simulink model "ThrustVectorControlModelRocket"  (R2018a)
settings: Solver=FixedStepAuto  StartTime=0.0  StopTime=3.5  FixedStep=0.02  RelTol=1e-3
libraries: simulink_extras x7, simulink x5, sharedtransform x1, aerolibutil x1
settings Model: Creator=Doe  LastModifiedBy=rahul
settings OptimizationCC: DefaultParameterBehavior=Inlined  UseDivisionForNetSlopeComputation=on  UseFloatMulNetSlope=on  InlineInvariantSignals=on  PassReuseOutputArgsAs=Individual arguments  ZeroExternalMemoryAtStartup=off  ZeroInternalMemoryAtStartup=off  NoFixptDivByZeroProtection=on  EfficientFloat2IntCast=on  LifeSpan=1  OptimizeBlockOrder=speed  DifferentSizesBufferReuse=on
settings DebuggingCC: ParameterTunabilityLossMsg=error
settings HardwareCC: ProdBitPerInt=16  ProdBitPerPointer=16  ProdBitPerSizeT=16  ProdBitPerPtrDiffT=16  ProdLargestAtomicFloat=None  ProdWordSize=16  ProdLongLongMode=on  ProdHWDeviceType=Atmel->AVR (8-bit)
settings SFSimCC: MATLABDynamicMemAlloc=off
settings RTWCC: SystemTargetFile=ert.tlc  TemplateMakefile=ert_default_tmf  GenerateReport=on  IncludeHyperlinkInReport=on  LaunchReport=on  TargetLang=C++  GenerateTraceInfo=on  GenerateTraceReport=on  GenerateTraceReportSl=on  GenerateTraceReportSf=on  GenerateTraceReportEml=on
settings CodeAppCC: ForceParamTrailComments=on  IgnoreCustomStorageClasses=off  OperatorAnnotations=on  SimulinkDataObjDesc=on  SFDataObjDesc=on  CustomSymbolStrGlobalVar=rt$N$M  CustomSymbolStrType=$N$M  CustomSymbolStrFcn=$N$M$F  CustomSymbolStrMacro=$N$M  InsertBlockDesc=on
settings ERTTargetCC: TargetLangStandard=C++03 (ISO)  GenerateSampleERTMain=on  IncludeMdlTerminateFcn=off  CombineSignalStateStructs=on  MultiInstanceERTCode=on  CodeInterfacePackaging=C++ class  SupportComplex=off  SupportContinuousTime=on  InlinedParameterPlacement=NonHierarchical  RootIOFormat=Structure reference  ERTCustomFileTemplate=example_file_process.tlc  ERTFilePackagingFormat=CompactWithDataFile

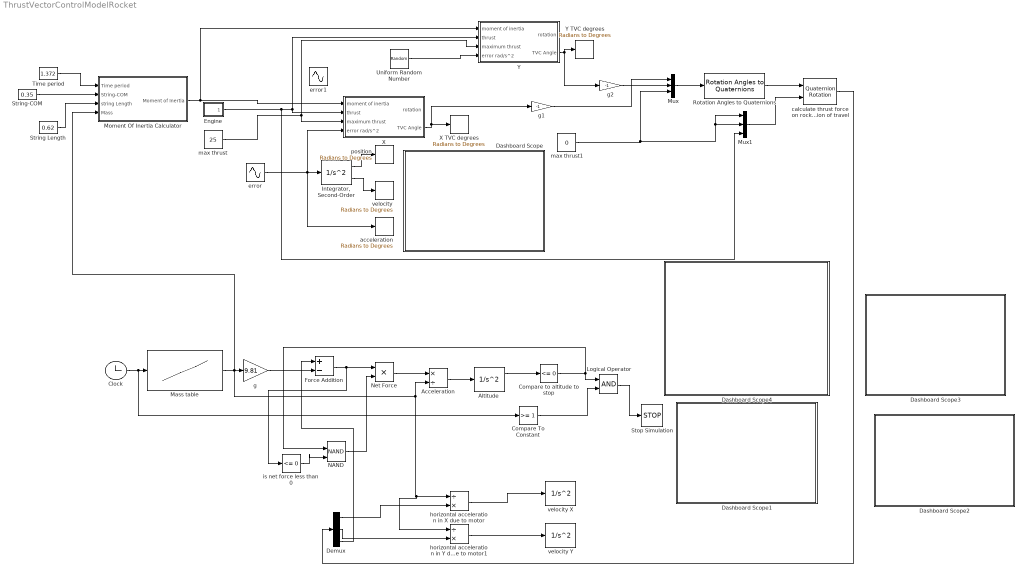
== system ThrustVectorControlModelRocket ==
  Acceleration : Product  Inputs=*/
  Altitude : SecondOrderIntegrator
  Clock : Clock
  Compare To Constant : simulink/Logic and Bit Operations/Compare To Constant  relop=>=  const=1  OutDataTypeStr=boolean
  Compare to altitude to stop : simulink/Logic and Bit Operations/Compare To Constant  relop=<=  const=0  OutDataTypeStr=boolean
  Dashboard Scope : Subsystem  DialogController=hmiCreateDDGDialog  IsWebBlock=on  mask(MWDashboardBlock){webBlockId=e89a2d5a-8c4b-4126-bd68-68e024a85c17, webBlockType=sdiscope, ShowInitialText=on, HMISrcModelName=ThrustVectorControlModelRocket}
      mask prompts: webBlockId "WebBlock Id"; webBlockType "WebBlock Type"; HMISrcModelName "Source Model"
      mask help: SimulinkHMI:dialogs:HMIScopeDialogDesc
      mask Help: helpview([docroot '/mapfiles/simulink.map'], 'hmi_scope')
      mask Display:
      | if strcmp(get_param(bdroot(gcb),'BlockDiagramType'), 'library')
      |     image([(matlabroot) '/toolbox/simulink/hmi/icons/DashboardScope.png']);
      | end
  Dashboard Scope1 : Subsystem  DialogController=hmiCreateDDGDialog  IsWebBlock=on  mask(MWDashboardBlock){webBlockId=79388a0e-acf4-4a0f-9f6d-7a65b6fe74ae, webBlockType=sdiscope, ShowInitialText=on, HMISrcModelName=ThrustVectorControlModelRocket}
      mask prompts: webBlockId "WebBlock Id"; webBlockType "WebBlock Type"; HMISrcModelName "Source Model"
      mask help: SimulinkHMI:dialogs:HMIScopeDialogDesc
      mask Help: helpview([docroot '/mapfiles/simulink.map'], 'hmi_scope')
      mask Display:
      | if strcmp(get_param(bdroot(gcb),'BlockDiagramType'), 'library')
      |     image([(matlabroot) '/toolbox/simulink/hmi/icons/DashboardScope.png']);
      | end
  Dashboard Scope2 : Subsystem  DialogController=hmiCreateDDGDialog  IsWebBlock=on  mask(MWDashboardBlock){webBlockId=9be5d186-43fb-46f6-9404-6296feed70e7, webBlockType=sdiscope, ShowInitialText=on, HMISrcModelName=ThrustVectorControlModelRocket}
      mask prompts: webBlockId "WebBlock Id"; webBlockType "WebBlock Type"; HMISrcModelName "Source Model"
      mask help: SimulinkHMI:dialogs:HMIScopeDialogDesc
      mask Help: helpview([docroot '/mapfiles/simulink.map'], 'hmi_scope')
      mask Display:
      | if strcmp(get_param(bdroot(gcb),'BlockDiagramType'), 'library')
      |     image([(matlabroot) '/toolbox/simulink/hmi/icons/DashboardScope.png']);
      | end
  Dashboard Scope3 : Subsystem  DialogController=hmiCreateDDGDialog  IsWebBlock=on  mask(MWDashboardBlock){webBlockId=200297c4-bc4f-4d0c-b2fb-30ef607173bc, webBlockType=sdiscope, ShowInitialText=on, HMISrcModelName=ThrustVectorControlModelRocket}
      mask prompts: webBlockId "WebBlock Id"; webBlockType "WebBlock Type"; HMISrcModelName "Source Model"
      mask help: SimulinkHMI:dialogs:HMIScopeDialogDesc
      mask Help: helpview([docroot '/mapfiles/simulink.map'], 'hmi_scope')
      mask Display:
      | if strcmp(get_param(bdroot(gcb),'BlockDiagramType'), 'library')
      |     image([(matlabroot) '/toolbox/simulink/hmi/icons/DashboardScope.png']);
      | end
  Dashboard Scope4 : Subsystem  DialogController=hmiCreateDDGDialog  IsWebBlock=on  mask(MWDashboardBlock){webBlockId=5d101f40-2dd7-4f18-8b35-aff23edb331a, webBlockType=sdiscope, ShowInitialText=on, HMISrcModelName=ThrustVectorControlModelRocket}
      mask prompts: webBlockId "WebBlock Id"; webBlockType "WebBlock Type"; HMISrcModelName "Source Model"
      mask help: SimulinkHMI:dialogs:HMIScopeDialogDesc
      mask Help: helpview([docroot '/mapfiles/simulink.map'], 'hmi_scope')
      mask Display:
      | if strcmp(get_param(bdroot(gcb),'BlockDiagramType'), 'library')
      |     image([(matlabroot) '/toolbox/simulink/hmi/icons/DashboardScope.png']);
      | end
  Demux : Demux  Outputs=3
  Engine : Subsystem
  Force Addition : Sum  Inputs=+-
  "Integrator, Second-Order" : SecondOrderIntegrator
  Logical Operator : Logic  AllPortsSameDT=off  OutDataTypeStr=boolean
  Mass table : Lookup  InputValues=[0,1]  Table=[0.975,.8]  LookUpMeth=Use Input Nearest  SaturateOnIntegerOverflow=on
  Moment Of Inertia Calculator : Subsystem
  Mux : Mux  Inputs=3
  Mux1 : Mux  Inputs=3
  NAND : Logic  Operator=NAND  IconShape=distinctive  AllPortsSameDT=off  OutDataTypeStr=boolean
  Net Force : Product  Inputs=**
  Rotation Angles to Quaternions : sharedtransform/Rotation Angles to Quaternions  rotationOrder=XYZ  aMode=aMode
      settings: SourceProductName=Aerospace Blockset  SourceProductBaseCode=AE
  Stop Simulation : Stop
  String Length : Constant  Value=0.62
  String-COM : Constant  Value=0.35
  Time period : Constant  Value=1.372
  Uniform Random Number : UniformRandomNumber  Minimum=-3  Maximum=3  SampleTime=.4
  X : Subsystem
  X TVC degrees : simulink_extras/Transformations/Radians to Degrees
  Y : Subsystem
  Y TVC degrees : simulink_extras/Transformations/Radians to Degrees
  acceleration : simulink_extras/Transformations/Radians to Degrees
  calculate thrust force on rocket in direction of travel : aerolibutil/Quaternion Rotation
  error : Sin  Amplitude=2  Frequency=2  SampleTime=0
  error1 : Sin  Frequency=4  SampleTime=0
  g : Gain  Gain=9.81
  g1 : Gain  Gain=-1
  g2 : Gain  Gain=-1
  horizontal acceleration in X due to motor : Product  Inputs=/*
  horizontal acceleration in Y due to motor1 : Product  Inputs=/*
  is net force less than 0 : simulink/Logic and Bit Operations/Compare To Constant  relop=<=  const=0  OutDataTypeStr=boolean
  max thrust : Constant  Value=25
  max thrust1 : Constant  Value=0
  position : simulink_extras/Transformations/Radians to Degrees
  velocity : simulink_extras/Transformations/Radians to Degrees
  velocity X : SecondOrderIntegrator
  velocity Y : SecondOrderIntegrator
  wires:
  String-COM/1 -> Moment Of Inertia Calculator/2(String-COM)
  Time period/1 -> Moment Of Inertia Calculator/1(Time period)
  String Length/1 -> Moment Of Inertia Calculator/3(string Length)
  NAND/1 -> Net Force/2
  Acceleration/1 -> Altitude/1
  Force Addition/1 -> is net force less than 0/1, Net Force/1
  Clock/1 -> Compare To Constant/1, Mass table/1
  Net Force/1 -> Acceleration/1
  Mass table/1 -> g/1, Acceleration/2, horizontal acceleration in Y due to motor1/1, horizontal acceleration in X due to motor/1, Moment Of Inertia Calculator/4(Mass)
  g/1 -> Force Addition/2
  is net force less than 0/1 -> NAND/2
  Altitude/1 -> Compare to altitude to stop/1
  Compare To Constant/1 -> Logical Operator/2
  Compare to altitude to stop/1 -> Logical Operator/1, NAND/1
  error/1 -> X/4(error rad/s^2), acceleration/1, "Integrator, Second-Order"/1
  Moment Of Inertia Calculator/1(Moment of Inertia) -> Y/1(moment of inertia), X/1(moment of inertia)
  max thrust/1 -> Y/3(maximum thrust), X/3(maximum thrust)
  "Integrator, Second-Order"/1 -> position/1
  "Integrator, Second-Order"/2 -> velocity/1
  X/2(TVC Angle) -> g1/1, X TVC degrees/1
  Mux/1 -> Rotation Angles to Quaternions/1
  Rotation Angles to Quaternions/1 -> calculate thrust force on rocket in direction of travel/1
  Mux1/1 -> calculate thrust force on rocket in direction of travel/2
  Logical Operator/1 -> Stop Simulation/1
  calculate thrust force on rocket in direction of travel/1 -> Demux/1
  g2/1 -> Mux/2
  max thrust1/1 -> Mux1/1, Mux1/2, Mux/3
  Y/2(TVC Angle) -> Y TVC degrees/1, g2/1
  g1/1 -> Mux/1
  Uniform Random Number/1 -> Y/4(error rad/s^2)
  Engine/1(Thrust) -> Mux1/3, Y/2(thrust), X/2(thrust)
  Demux/1 -> horizontal acceleration in X due to motor/2
  horizontal acceleration in X due to motor/1 -> velocity X/1
  Demux/3 -> Force Addition/1
  horizontal acceleration in Y due to motor1/1 -> velocity Y/1
  Demux/2 -> horizontal acceleration in Y due to motor1/2

== system ThrustVectorControlModelRocket/Dashboard Scope ==

== system ThrustVectorControlModelRocket/Dashboard Scope1 ==

== system ThrustVectorControlModelRocket/Dashboard Scope2 ==

== system ThrustVectorControlModelRocket/Dashboard Scope3 ==

== system ThrustVectorControlModelRocket/Dashboard Scope4 ==

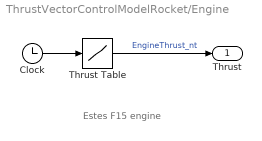
== system ThrustVectorControlModelRocket/Engine ==
  note: Estes F15 engine
  Clock : Clock
  Thrust Table : Lookup  InputValues=|  Table=[0,12.5,25,16.5,15.25,15,14.5,14.5,14.25,14,13,13,0]  LookUpMeth=Interpolation-Use End Values  SaturateOnIntegerOverflow=on
      | [0,
      | 0.25,
      | 0.5,
      | 0.75,
      | 1,
      | 1.25,
      | 1.5,
      | 2,
      | 2.25,
      | 2.5,
      | 3,
      | 3.25,
      | 3.5]
  Thrust : Outport
  wires:
  Clock/1 -> Thrust Table/1
  Thrust Table/1 -> Thrust/1  "EngineThrust_nt"

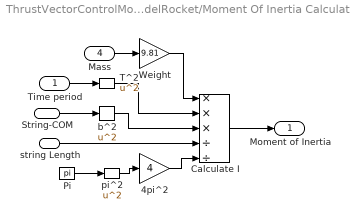
== system ThrustVectorControlModelRocket/Moment Of Inertia Calculator ==
  Time period : Inport
  String-COM : Inport  Port=2
  string Length : Inport  Port=3
  Mass : Inport  Port=4
  4pi^2 : Gain  Gain=4
  Calculate I : Product  Inputs=***//
  Pi : Constant  Value=pi
  T^2 : Math  Operator=square  SaturateOnIntegerOverflow=on
  Weight : Gain  Gain=9.81
  b^2 : Math  Operator=square  SaturateOnIntegerOverflow=on
  pi^2 : Math  Operator=square  SaturateOnIntegerOverflow=on
  Moment of Inertia : Outport
  wires:
  Time period/1 -> T^2/1
  Calculate I/1 -> Moment of Inertia/1
  string Length/1 -> Calculate I/4
  Mass/1 -> Weight/1
  Weight/1 -> Calculate I/1
  pi^2/1 -> 4pi^2/1
  b^2/1 -> Calculate I/3
  T^2/1 -> Calculate I/2
  String-COM/1 -> b^2/1
  Pi/1 -> pi^2/1
  4pi^2/1 -> Calculate I/5

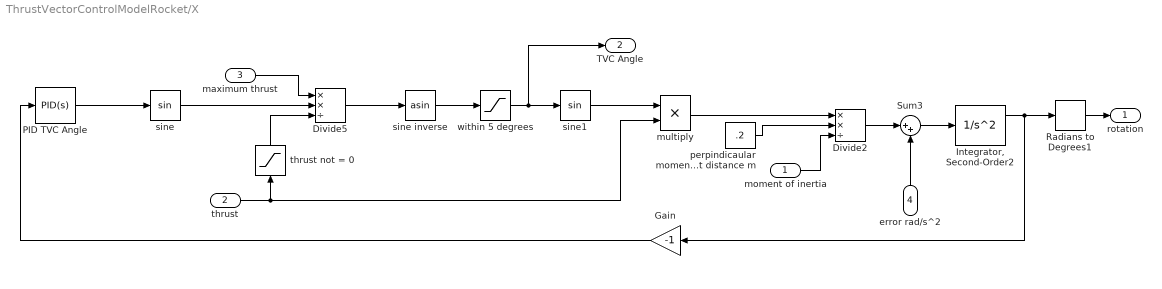
== system ThrustVectorControlModelRocket/X ==
  moment of inertia : Inport
  thrust : Inport  Port=2
  maximum thrust : Inport  Port=3
  error rad/s^2 : Inport  Port=4
  Divide2 : Product  Inputs=**/
  Divide5 : Product  Inputs=**/
  Gain : Gain  Gain=-1
  "Integrator, Second-Order2" : SecondOrderIntegrator
  PID TVC Angle : simulink/Continuous/PID Controller  Controller=PID  TimeDomain=Continuous-time  SampleTime=-1  IntegratorMethod=Forward Euler  FilterMethod=Forward Euler  Form=Parallel  UseFilter=on  ControllerParametersSource=internal  P=0.382662534441352  I=0.206393482611663  D=0.139903294226043  N=36.46824066771  InitialConditionSource=internal  InitialConditionForIntegrator=0  InitialConditionForFilter=0  ExternalReset=none  LimitOutput=on  UpperSaturationLimit=0.08726646  LowerSaturationLimit=-0.08726646  LinearizeAsGain=on  AntiWindupMode=none  Kb=1  TrackingMode=off  Kt=1  PParamMin=[]  PParamMax=[]  IParamMin=[]  IParamMax=[]  DParamMin=[]  DParamMax=[]  NParamMin=[]  NParamMax=[]  KbParamMin=[]  KbParamMax=[]  KtParamMin=[]  KtParamMax=[]  POutMin=[]  POutMax=[]  IOutMin=[]  IOutMax=[]  DOutMin=[]  DOutMax=[]  NOutMin=[]  NOutMax=[]  KbOutMin=[]  KbOutMax=[]  KtOutMin=[]  KtOutMax=[]  IntegratorOutMin=[]  IntegratorOutMax=[]  FilterOutMin=[]  FilterOutMax=[]  SumOutMin=[]  SumOutMax=[]  SumI1OutMin=[]  SumI1OutMax=[]  SumI2OutMin=[]  SumI2OutMax=[]  SumI3OutMin=[]  SumI3OutMax=[]  SumDOutMin=[]  SumDOutMax=[]  SaturationOutMin=[]  SaturationOutMax=[]  IntegratorContinuousStateAttributes=''  IntegratorStateMustResolveToSignalObject=off  IntegratorRTWStateStorageClass=Auto  FilterContinuousStateAttributes=''  FilterStateMustResolveToSignalObject=off  FilterRTWStateStorageClass=Auto  DifferentiatorICPrevScaledInput=0  DifferentiatorOutMin=[]  DifferentiatorOutMax=[]  FilterDiffOutCoefMin=[]  FilterDiffOutCoefMax=[]  SumDenOutMin=[]  SumDenOutMax=[]  SumNumOutMin=[]  SumNumOutMax=[]  ReciprocalOutMin=[]  ReciprocalOutMax=[]  DivideOutMin=[]  DivideOutMax=[]  TunerSelectOption=Transfer Function Based (PID Tuner App)
  Radians to Degrees1 : simulink_extras/Transformations/Radians to Degrees
  Sum3 : Sum  Inputs=|++
  multiply : Product  Inputs=**
  perpindicaular moment distance m : Constant  Value=.2
  sine : Trigonometry
  sine inverse : Trigonometry  Operator=asin
  sine1 : Trigonometry
  thrust not = 0 : Saturate  UpperLimit=100  LowerLimit=.001
  within 5 degrees : Saturate  UpperLimit=0.08726646  LowerLimit=-0.08726646
  rotation : Outport
  TVC Angle : Outport  Port=2
  wires:
  error rad/s^2/1 -> Sum3/2
  perpindicaular moment distance m/1 -> Divide2/2
  Divide5/1 -> sine inverse/1
  sine inverse/1 -> within 5 degrees/1
  "Integrator, Second-Order2"/1 -> Radians to Degrees1/1, Gain/1
  Sum3/1 -> "Integrator, Second-Order2"/1
  moment of inertia/1 -> Divide2/3
  Divide2/1 -> Sum3/1
  sine/1 -> Divide5/2
  PID TVC Angle/1 -> sine/1
  multiply/1 -> Divide2/1
  thrust not = 0/1 -> Divide5/3
  maximum thrust/1 -> Divide5/1
  thrust/1 -> multiply/2, thrust not = 0/1
  sine1/1 -> multiply/1
  within 5 degrees/1 -> sine1/1, TVC Angle/1
  Gain/1 -> PID TVC Angle/1
  Radians to Degrees1/1 -> rotation/1

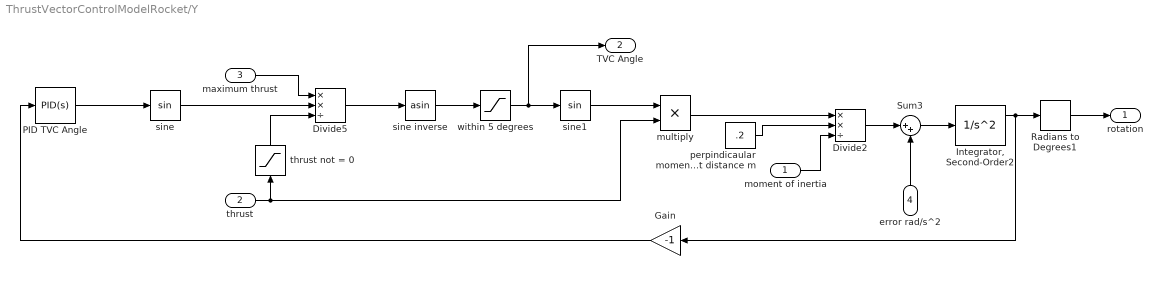
== system ThrustVectorControlModelRocket/Y ==
  moment of inertia : Inport
  thrust : Inport  Port=2
  maximum thrust : Inport  Port=3
  error rad/s^2 : Inport  Port=4
  Divide2 : Product  Inputs=**/
  Divide5 : Product  Inputs=**/
  Gain : Gain  Gain=-1
  "Integrator, Second-Order2" : SecondOrderIntegrator
  PID TVC Angle : simulink/Continuous/PID Controller  Controller=PID  TimeDomain=Continuous-time  SampleTime=-1  IntegratorMethod=Forward Euler  FilterMethod=Forward Euler  Form=Parallel  UseFilter=on  ControllerParametersSource=internal  P=0.382662534441352  I=0.206393482611663  D=0.139903294226043  N=36.46824066771  InitialConditionSource=internal  InitialConditionForIntegrator=0  InitialConditionForFilter=0  ExternalReset=none  LimitOutput=on  UpperSaturationLimit=0.08726646  LowerSaturationLimit=-0.08726646  LinearizeAsGain=on  AntiWindupMode=none  Kb=1  TrackingMode=off  Kt=1  PParamMin=[]  PParamMax=[]  IParamMin=[]  IParamMax=[]  DParamMin=[]  DParamMax=[]  NParamMin=[]  NParamMax=[]  KbParamMin=[]  KbParamMax=[]  KtParamMin=[]  KtParamMax=[]  POutMin=[]  POutMax=[]  IOutMin=[]  IOutMax=[]  DOutMin=[]  DOutMax=[]  NOutMin=[]  NOutMax=[]  KbOutMin=[]  KbOutMax=[]  KtOutMin=[]  KtOutMax=[]  IntegratorOutMin=[]  IntegratorOutMax=[]  FilterOutMin=[]  FilterOutMax=[]  SumOutMin=[]  SumOutMax=[]  SumI1OutMin=[]  SumI1OutMax=[]  SumI2OutMin=[]  SumI2OutMax=[]  SumI3OutMin=[]  SumI3OutMax=[]  SumDOutMin=[]  SumDOutMax=[]  SaturationOutMin=[]  SaturationOutMax=[]  IntegratorContinuousStateAttributes=''  IntegratorStateMustResolveToSignalObject=off  IntegratorRTWStateStorageClass=Auto  FilterContinuousStateAttributes=''  FilterStateMustResolveToSignalObject=off  FilterRTWStateStorageClass=Auto  DifferentiatorICPrevScaledInput=0  DifferentiatorOutMin=[]  DifferentiatorOutMax=[]  FilterDiffOutCoefMin=[]  FilterDiffOutCoefMax=[]  SumDenOutMin=[]  SumDenOutMax=[]  SumNumOutMin=[]  SumNumOutMax=[]  ReciprocalOutMin=[]  ReciprocalOutMax=[]  DivideOutMin=[]  DivideOutMax=[]  TunerSelectOption=Transfer Function Based (PID Tuner App)
  Radians to Degrees1 : simulink_extras/Transformations/Radians to Degrees
  Sum3 : Sum  Inputs=|++
  multiply : Product  Inputs=**
  perpindicaular moment distance m : Constant  Value=.2
  sine : Trigonometry
  sine inverse : Trigonometry  Operator=asin
  sine1 : Trigonometry
  thrust not = 0 : Saturate  UpperLimit=100  LowerLimit=.001
  within 5 degrees : Saturate  UpperLimit=0.08726646  LowerLimit=-0.08726646
  rotation : Outport
  TVC Angle : Outport  Port=2
  wires:
  error rad/s^2/1 -> Sum3/2
  perpindicaular moment distance m/1 -> Divide2/2
  Divide5/1 -> sine inverse/1
  sine inverse/1 -> within 5 degrees/1
  Sum3/1 -> "Integrator, Second-Order2"/1
  moment of inertia/1 -> Divide2/3
  Divide2/1 -> Sum3/1
  sine/1 -> Divide5/2
  PID TVC Angle/1 -> sine/1
  multiply/1 -> Divide2/1
  thrust not = 0/1 -> Divide5/3
  maximum thrust/1 -> Divide5/1
  thrust/1 -> multiply/2, thrust not = 0/1
  sine1/1 -> multiply/1
  within 5 degrees/1 -> sine1/1, TVC Angle/1
  Gain/1 -> PID TVC Angle/1
  Radians to Degrees1/1 -> rotation/1
  "Integrator, Second-Order2"/1 -> Gain/1, Radians to Degrees1/1
